simulink model "q_torsion_id"  (R2024a)
settings: Solver=FixedStepDiscrete  StartTime=0.0  StopTime=5  FixedStep=0.002  RelTol=1e-3  EnableMultiTasking=on
values from neighbouring files (symbols this model uses):
  K_AMP = 1    [setup_torsion.m]
  K_ENC = 0    [config_srv02.m]
  VMAX_AMP = 0    [config_srv02.m]
  VMAX_DAC = 10    [setup_torsion.m]
undefined symbols (not defined in the file or in its folder): HIL, qc_get_step_size
libraries: quarc_library x3, simulink_extras x2
settings Model: SimulationMode=external  ExtModeTrigDuration=10000  Creator=MLevis  LastModifiedBy=quarc_user
settings SolverCC: AlgebraicLoopSolver=TrustRegion  PositivePriorityOrder=on
settings DataIOCC: LimitDataPoints=on  SaveFormat=Array  SignalLoggingSaveFormat=ModelDataLogs  ReturnWorkspaceOutputs=off
settings OptimizationCC: ExpressionDepthLimit=2147483647  InitFltsAndDblsToZero=on
settings DebuggingCC: SaveWithParameterizedLinksMsg=none  UnderspecifiedInitializationDetection=Classic  MergeDetectMultiDrivingBlocksExec=none  SolverPrmCheckMsg=warning  FcnCallInpInsideContextMsg=warning  UnconnectedInputMsg=warning  UnconnectedOutputMsg=warning  UnconnectedLineMsg=warning  StateNameClashWarn=warning  SFUnexpectedBacktrackingDiag=warning  SFNoUnconditionalDefaultTransitionDiag=warning  SFExecutionAtInitializationDiag=none  ArithmeticOperatorsInVariantConditions=warning
settings ModelReferenceCC: PropagateSignalLabelsOutOfModel=off
settings SFSimCC: SimUseLocalCustomCode=off  CustomCodeUndefinedFunction=UseInterfaceOnly
settings RTWCC: Description=QUARC Win64 Target Using Toolchain  SystemTargetFile=quarc_win64.tlc  TemplateMakefile=quarc_default_tmf  RTWUseLocalCustomCode=off  Toolchain=QUARC win64 | nmake (64-bit Windows)  BuildConfiguration=Faster Runs  GPUComputeCapability=3.5
settings CodeAppCC: StateflowObjectComments=on
settings STFCustomTargetCC: TargetLangStandard=C89/C90 (ANSI)  ConcurrentExecutionCompliant=on  SystemTargetFile=quarc_win64.tlc
settings GRTTargetCC: TargetLangStandard=C89/C90 (ANSI)  ParMdlRefBuildCompliant=off  CompOptLevelCompliant=off  CombineOutputUpdateFcns=off  MatFileLogging=off  CPPClassGenCompliant=off  GRTInterface=on  ExtMode=on  ExtModeMexFile=quarc_comm
settings ConfigComp: CovMetricSettings=dw  CovSaveCumulativeToWorkspaceVar=on  CovSaveSingleToWorkspaceVar=on  CovExternalEMLEnable=off

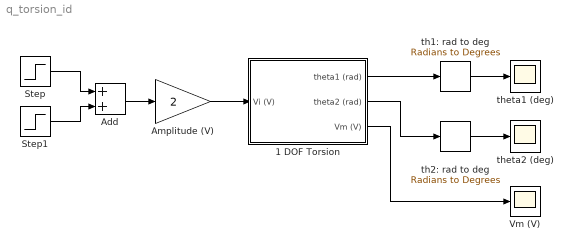
== system q_torsion_id ==
  1 DOF Torsion : Subsystem
  Add : Sum
  Amplitude (V) : Gain  Gain=2  SaturateOnIntegerOverflow=on  OutDataTypeStr=Inherit: Same as input  ParamDataTypeStr=Inherit: Same as input
  Step : Step  SampleTime=0
  Step1 : Step  Time=1.1  After=-1  SampleTime=0
  Vm (V) : Scope
  th1: rad to deg : simulink_extras/Transformations/Radians to Degrees
  th2: rad to deg : simulink_extras/Transformations/Radians to Degrees
  theta1 (deg) : Scope
  theta2 (deg) : Scope
  wires:
  1 DOF Torsion/1(theta1 (rad)) -> th1: rad to deg/1
  1 DOF Torsion/2(theta2 (rad)) -> th2: rad to deg/1
  th2: rad to deg/1 -> theta2 (deg)/1
  1 DOF Torsion/3(Vm (V)) -> Vm (V)/1
  Amplitude (V)/1 -> 1 DOF Torsion/1(Vi (V))
  th1: rad to deg/1 -> theta1 (deg)/1
  Step/1 -> Add/1
  Step1/1 -> Add/2
  Add/1 -> Amplitude (V)/1

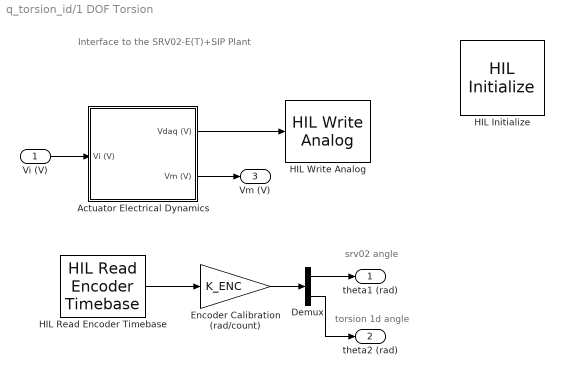
== system q_torsion_id/1 DOF Torsion ==
  note: Interface to the SRV02-E(T)+SIP Plant
  note: srv02 angle
  note: torsion 1d angle
  Vi (V) : Inport
  Actuator Electrical Dynamics : Subsystem
  Demux : Demux  Outputs=2
  Encoder Calibration (rad/count) : Gain  Gain=K_ENC  SaturateOnIntegerOverflow=on  OutDataTypeStr=Inherit: Same as input  ParamDataTypeStr=Inherit: Same as input
  HIL Initialize : quarc_library/Data Acquisition/Generic/Configuration/HIL Initialize  object_name=HIL-1  board_type=q2_usb  board_number=0  board_options=d0=digital;d1=digital;led=auto;update_rate=normal  exclusive=off  active=off  hardware_clocks=[0:2]  clock_modes=[]  initial_clock_frequencies=[]  set_clock_params_at_start=off  set_clock_params_at_switch_in=off  set_clock_frequencies_at_start=off  set_clock_frequencies_at_switch_in=off  analog_input_channels=[0:1]  analog_input_maximums=10  analog_input_minimums=-10  set_analog_input_params_at_start=on  set_analog_input_params_at_switch_in=off  analog_output_channels=[0:1]  analog_output_maximums=10  analog_output_minimums=-10  initial_analog_outputs=[0]  final_analog_outputs=[0]  watchdog_analog_outputs=0  set_analog_output_params_at_start=on  set_analog_output_params_at_switch_in=off  set_analog_outputs_at_start=on  set_analog_outputs_at_switch_in=off  set_analog_outputs_at_terminate=on  set_analog_outputs_at_switch_out=off  set_analog_outputs_on_watchdog=on  digital_input_channels=[]  digital_output_channels=[0:7]  digital_output_configuration=[]  initial_digital_outputs=[0]  final_digital_outputs=[0]  watchdog_digital_outputs=[0]  set_digital_output_params_at_start=off  set_digital_output_params_at_switch_in=off  set_digital_outputs_at_start=on  set_digital_outputs_at_switch_in=off  set_digital_outputs_at_terminate=on  set_digital_outputs_at_switch_out=off  set_digital_outputs_on_watchdog=on  encoder_channels=[0:1]  quadrature=[4]  encoder_filter_frequency=[]  initial_encoder_counts=[0]  set_encoder_params_at_start=on  set_encoder_params_at_switch_in=off  set_encoder_counts_at_start=on  set_encoder_counts_at_switch_in=off  pwm_channels=[]  pwm_modes=[0]  pwm_frequency=1/0.020  pwm_configuration=[]  pwm_alignment=[]  pwm_polarity=[]  pwm_leading_deadband=[]  pwm_trailing_deadband=[]  initial_pwm_outputs=[0]  final_pwm_outputs=[0]  watchdog_pwm_outputs=[0]  set_pwm_params_at_start=on  set_pwm_params_at_switch_in=off  set_pwm_outputs_at_start=on  set_pwm_outputs_at_switch_in=off  set_pwm_outputs_at_terminate=on  set_pwm_outputs_at_switch_out=off  set_pwm_outputs_on_watchdog=off  other_output_channels=[]  initial_other_outputs=[]  final_other_outputs=[]  watchdog_other_outputs=[]  set_other_outputs_at_start=off  set_other_outputs_at_switch_in=off  set_other_outputs_at_terminate=off  set_other_outputs_at_switch_out=off  set_other_outputs_on_watchdog=off
  HIL Read Encoder Timebase : quarc_library/Data Acquisition/Generic/Timebases/HIL Read Encoder Timebase  object_name=HIL-1  clock=0  channels=[0:1]  samples_in_buffer=max(ceil(1/qc_get_step_size), 1)  active=on  vector_output=on  data_type_mode=Inherit via back propagation  data_type=double
  HIL Write Analog : quarc_library/Data Acquisition/Generic/Immediate I//O/HIL Write Analog  object_name=HIL-1  channels=0  sample_time=-1  active=off  vector_input=off
  theta1 (rad) : Outport
  theta2 (rad) : Outport  Port=2
  Vm (V) : Outport  Port=3
  wires:
  Actuator Electrical Dynamics/1(Vdaq (V)) -> HIL Write Analog/1
  Actuator Electrical Dynamics/2(Vm (V)) -> Vm (V)/1
  HIL Read Encoder Timebase/1 -> Encoder Calibration (rad/count)/1
  Vi (V)/1 -> Actuator Electrical Dynamics/1(Vi (V))
  Encoder Calibration (rad/count)/1 -> Demux/1
  Demux/1 -> theta1 (rad)/1
  Demux/2 -> theta2 (rad)/1

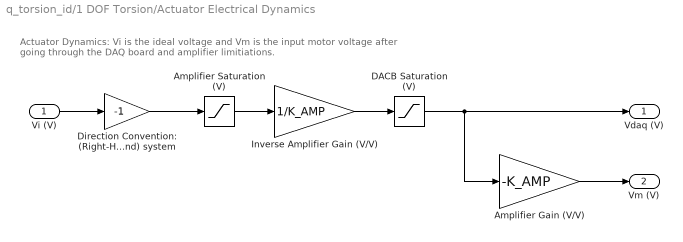
== system q_torsion_id/1 DOF Torsion/Actuator Electrical Dynamics ==
  note: Actuator Dynamics: Vi is the ideal voltage and Vm is the
      | input motor voltage after going through the DAQ board and amplifier limitiations.
  Vi (V) : Inport
  Amplifier Gain (V/V) : Gain  Gain=-K_AMP
  Amplifier Saturation (V) : Saturate  UpperLimit=VMAX_AMP  LowerLimit=-VMAX_AMP
  DACB Saturation (V) : Saturate  UpperLimit=VMAX_DAC  LowerLimit=-VMAX_DAC
  Direction Convention: (Right-Hand) system : Gain  Gain=-1  SaturateOnIntegerOverflow=on  OutDataTypeStr=Inherit: Same as input  ParamDataTypeStr=Inherit: Same as input
  Inverse Amplifier Gain (V/V) : Gain  Gain=1/K_AMP
  Vdaq (V) : Outport
  Vm (V) : Outport  Port=2
  wires:
  Direction Convention: (Right-Hand) system/1 -> Amplifier Saturation (V)/1
  Amplifier Gain (V/V)/1 -> Vm (V)/1
  DACB Saturation (V)/1 -> Vdaq (V)/1, Amplifier Gain (V/V)/1
  Inverse Amplifier Gain (V/V)/1 -> DACB Saturation (V)/1
  Vi (V)/1 -> Direction Convention: (Right-Hand) system/1
  Amplifier Saturation (V)/1 -> Inverse Amplifier Gain (V/V)/1
